simulink model "StateFlow_4"  (R2018a)
settings: Solver=VariableStepAuto  StartTime=0.0  StopTime=10.0  RelTol=1e-3
settings Model: Creator=Choaib ELMADI  LastModifiedBy=Choaib ELMADI

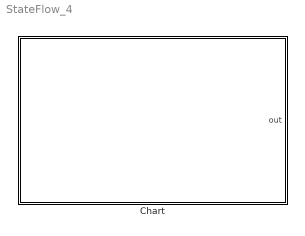
== system StateFlow_4 ==
  Chart : Stateflow chart  TreatAsAtomicUnit=on

== stateflow chart StateFlow_4/Chart ==
  note: Do not put any code along
      | the transitions that run
      | down the right side!
  (default) -> (junction 60) [order 1] : % For Loop Pattern
  (junction 61) -> (junction 59) [order 1] : [i<10]
  (junction 59) -> (junction 62) : {out=i;}
  (default) -> (junction 42) [order 2] : % Switch Case Pattern
  (default) -> (junction 17) [order 3] : % IF Pattern
  (junction 60) -> (junction 61) : {i=0;}
  (junction 17) -> (junction 18) [order 1] : [in==1]
  (junction 42) -> (junction 43) [order 1] : [in == 0]
  (junction 17) -> (junction 19) [order 2]
  (junction 18) -> (junction 26) : {out=1;}
  (junction 62) -> (junction 61) : {i=i+1;}
  (junction 42) -> (junction 46) [order 2]
  (junction 43) -> (junction 44) : {out=0;}
  (junction 61) -> (junction 63) [order 2]
  (junction 19) -> (junction 20) [order 1] : [in==0]
  (junction 44) -> (junction 45)
  (junction 19) -> (junction 21) [order 2]
  (junction 20) -> (junction 25) : {out=0;}
  (junction 45) -> (junction 49)
  (junction 46) -> (junction 47) [order 1] : [in == 1]
  (junction 46) -> (junction 50) [order 2] : {out=9;}
  (junction 47) -> (junction 48) : {out=1;}
  (junction 21) -> (junction 22) [order 1] : [in==2]
  (junction 21) -> (junction 23) [order 2] : {out=9;}
  (junction 22) -> (junction 24) : {out=2;}
  (default) -> (junction 70) [order 4] : % While Pattern
  (junction 48) -> (junction 49)
  (junction 49) -> (junction 51)
  (junction 24) -> (junction 23)
  (junction 25) -> (junction 24)
  (junction 26) -> (junction 25)
  (junction 70) -> (junction 72)
  (junction 23) -> (junction 27)
  (junction 72) -> (junction 71) [order 1] : [i<10]
  (junction 71) -> (junction 73) : {out=i;}
  (junction 51) -> (junction 50)
  (junction 50) -> (junction 52)
  (junction 73) -> (junction 72)
  (junction 72) -> (junction 74) [order 2]
  data: out output double; i local double
